simulink model "mpc_model_dual_module_tobecombined"  (R2019a)
settings: Solver=FixedStepAuto  StartTime=0.0  StopTime=Tfinal  RelTol=1e-3
values from neighbouring files (symbols this model uses):
  A = [-0.0285 -0.0014; -0.0371 -0.1476]    [model.m]
  DCLINK_Cap = 1000e-12    (= 1e-09)    [mpc_model_parameters.m]    (also in mpc_model_parameters_dual_module.m = 0.001)
  FluxPM = MeanInducedVoltagePeak/(2*pi*100)    [mpc_model_parameters.m]    (also in mpc_model_parameters_dual_module.m)
  Inertia = 1e-2    (= 0.01)    [mpc_model_parameters.m]    (also in mpc_model_parameters_dual_module.m)
  iqrated = Trated/(1.5*PolePairs*FluxPM)    [mpc_model_parameters.m]    (also in mpc_model_parameters_dual_module.m)
  Ls = 3.5e-3    (= 0.0035)    [MPC_id_iq.m]    (also in mpc_model_parameters.m = 0.00351; mpc_model_parameters_dual_module.m = 0.00343)
  M1_FaultTime = 0.25    [mpc_model_parameters_dual_module.m]
  M2_FaultTime = 20    [mpc_model_parameters_dual_module.m]
  MeanLd = (1/12)*(Module1Phase_A_Ld+Module1Phase_B_Ld+Module1Phase_C_Ld+     Module2Phase_A_Ld+Module2Phase_B_Ld+Module2Phase_C_Ld+     Module3Phase_A_Ld+Module3Phase_B_Ld+Module3Phase_C_Ld+     Module4Phase_A_Ld+Module4Phase_B_Ld+Module4Phase_C_Ld)    [mpc_model_parameters.m]    (also in mpc_model_parameters_dual_module.m)
  MeanLq = (1/12)*(Module1Phase_A_Lq+Module1Phase_B_Lq+Module1Phase_C_Lq+     Module2Phase_A_Lq+Module2Phase_B_Lq+Module2Phase_C_Lq+     Module3Phase_A_Lq+Module3Phase_B_Lq+Module3Phase_C_Lq+     Module4Phase_A_Lq+Module4Phase_B_Lq+Module4Phase_C_Lq)    [mpc_model_parameters.m]    (also in mpc_model_parameters_dual_module.m)
  PolePairs = 10    [mpc_model_parameters.m]    (also in mpc_model_parameters_dual_module.m)
  Rin = 1e-3    (= 0.001)    [mpc_model_parameters.m]    (also in mpc_model_parameters_dual_module.m)
  Rs = 0.531    [Loss_Distribution.m]    (also in MPC_id_iq.m; mpc_model_parameters.m = 0.321; mpc_model_parameters_dual_module.m = 0.539)
  Sampling_time = 1e-6    (= 1e-06)    [mpc_model_parameters.m]    (also in mpc_model_parameters_dual_module.m)
  SpeedRef1 = 50    [mpc_model_parameters.m]    (also in mpc_model_parameters_dual_module.m = 35)
  SpeedRef2 = 100    [mpc_model_parameters.m]    (also in mpc_model_parameters_dual_module.m = 35)
  SpeedRefUpdateTime = 0.25    [mpc_model_parameters.m]    (also in mpc_model_parameters_dual_module.m = 1.75)
  Tload1 = 5    [mpc_model_parameters.m]    (also in mpc_model_parameters_dual_module.m = 30)
  Tload2 = 10    [mpc_model_parameters.m]    (also in mpc_model_parameters_dual_module.m = 63.6619772368)
  TloadUpdateTime = 0.5    [mpc_model_parameters.m]    (also in mpc_model_parameters_dual_module.m)
  Vdc = 50    [mpc_model_parameters.m]    (also in mpc_model_parameters_dual_module.m = 40)
  Vin = Vdc + Rin*(Pout/Vdc)    (= 50.04)    [mpc_model_parameters.m]    (also in mpc_model_parameters_dual_module.m = 40.05)
  ViscousFriction = 1e-3    (= 0.001)    [mpc_model_parameters.m]    (also in mpc_model_parameters_dual_module.m)
undefined symbols (not defined in the file or in its folder): DiscIntNeverNeededParam
libraries: powerlib x24, dspswit3 x13, fl_lib x5, simulink x3, powerlib_meascontrol x3, nesl_utility x3, sdl_lib x1, dspsigops x1
(part 2 of 2)

== matlab function mpc_model_dual_module_tobecombined/M1_prediction ==
  data: DutyA output; DutyB output; DutyC output; iqref input; idref input; IdMeasured input; IqMeasured input; Ls input; Rs input; PolePairs input; ShaftAngularSpeed input; FluxPM input; Vdc input; ElectricalAngle input; InterruptPulse input; DutyA_prev input; DutyB_prev input; DutyC_prev input; SimulationClock input; FaultOccuranceTime input; FswSelected_prev input; FswSelected output; IqRipplePrediction output; IqRipplePrediction_prev input
function [DutyA, DutyB, DutyC, FswSelected, IqRipplePrediction]  = fcn(iqref,idref,IdMeasured, IqMeasured, Ls, Rs,PolePairs,ShaftAngularSpeed,FluxPM,Vdc,ElectricalAngle,InterruptPulse,DutyA_prev, DutyB_prev, DutyC_prev, SimulationClock,FaultOccuranceTime,FswSelected_prev, IqRipplePrediction_prev)
Ld = Ls;
Lq = Ls;
I_Normalize = 11.7362; %this is the rated value of the IqMeasured
cost = zeros(1,8);
VdPrediction_1 = zeros(1,8);
VqPrediction_1 = zeros(1,8);
% FswOptions = [5000; 10000; 15000; 20000; 25000; 30000; 35000; 40000];
FswMax = 40000;
FswOptions = 1000:1000:FswMax;
cost = zeros(1,numel(FswOptions));
VdPrediction_1 = zeros(1,numel(FswOptions));
VqPrediction_1 = zeros(1,numel(FswOptions));
IqRipplePredictionArray = zeros(1,numel(FswOptions));
VoltageDuring_T1 = zeros(1,numel(FswOptions));
VoltageDuring_T2 = zeros(1,numel(FswOptions));
VoltageDuring_T0 = zeros(1,numel(FswOptions));
MagnitudePrediction_1 = zeros(1,numel(FswOptions));

SvpwmT1Prediction_1 =  zeros(1,numel(FswOptions));
SvpwmT2Prediction_1 =  zeros(1,numel(FswOptions));
SvpwmT0Prediction_1 =  zeros(1,numel(FswOptions));

ValfaPrediction_1 = zeros(1,numel(FswOptions)); 
VbetaPrediction_1 = zeros(1,numel(FswOptions)); 
maPrediction_1 = zeros(1,numel(FswOptions)); 

IqDelta_Prediction_During_T1_1 =  zeros(1,numel(FswOptions));
IqDelta_Prediction_During_T2_1 =  zeros(1,numel(FswOptions));
IqDelta_Prediction_During_T0_1 =  zeros(1,numel(FswOptions));
VoltageVectorAnglePredictionMod_1 = zeros(1,numel(FswOptions));
VoltageVectorAnglePrediction_1 = zeros(1,numel(FswOptions));

IqRippleCoeff = 10000;
IqRefCoeff = 100000;
IdRefCoeff = 15;
FswCoeff = 1500;
if(InterruptPulse==1)
    
    for i = 1:numel(FswOptions)
        % calculate vd vq
        VdPrediction_1(i) = Rs*IdMeasured + Ld*FswOptions(i)*(idref-IdMeasured)-PolePairs*ShaftAngularSpeed*Lq*IqMeasured;
        VqPrediction_1(i) = Rs*IqMeasured + Lq*FswOptions(i)*(iqref-IqMeasured)+PolePairs*ShaftAngularSpeed*(Ld*IdMeasured+FluxPM);
        
        MagnitudePrediction_1(i) = sqrt(VdPrediction_1(i)^2+VqPrediction_1(i)^2);
        
        ValfaPrediction_1(i) = sin(ElectricalAngle)*VdPrediction_1(i)+cos(ElectricalAngle)*VqPrediction_1(i);
        VbetaPrediction_1(i) =-cos(ElectricalAngle)*VdPrediction_1(i)+sin(ElectricalAngle)*VqPrediction_1(i);     
        
        VoltageVectorAnglePrediction_1(i) = atan2(VbetaPrediction_1(i),ValfaPrediction_1(i))+4*pi;
        VoltageVectorAnglePredictionMod_1(i) = mod(VoltageVectorAnglePrediction_1(i),pi/3);
        
        maPrediction_1(i) = MagnitudePrediction_1(i)/(Vdc/sqrt(3));
        

        
        if(SimulationClock>FaultOccuranceTime)
            SvpwmT1Prediction_1(i) = (1/FswOptions(i))*maPrediction_1(i)*sin(mod(VoltageVectorAnglePrediction_1(i),pi));
            SvpwmT2Prediction_1(i) = 0;
            SvpwmT0Prediction_1(i) = (1/FswOptions(i))-SvpwmT1Prediction_1(i)-SvpwmT2Prediction_1(i);       
%             IqRippleCoeff = 0;
%             FswCoeff = 1500;
        else
            SvpwmT1Prediction_1(i) = (1/FswOptions(i))*maPrediction_1(i)*sin(pi/3-VoltageVectorAnglePredictionMod_1(i));
            SvpwmT2Prediction_1(i) = (1/FswOptions(i))*maPrediction_1(i)*sin(VoltageVectorAnglePredictionMod_1(i));
            SvpwmT0Prediction_1(i) = (1/FswOptions(i))-SvpwmT1Prediction_1(i)-SvpwmT2Prediction_1(i);    
%             IqRippleCoeff = 10000;
%             FswCoeff = 1500;
        end        
        
        VoltageDuring_T1(i) = 2/3*Vdc-MagnitudePrediction_1(i);
        VoltageDuring_T2(i) = 2/3*Vdc-MagnitudePrediction_1(i);
        VoltageDuring_T0(i) = -MagnitudePrediction_1(i);
        
        IqDelta_Prediction_During_T1_1(i) = VoltageDuring_T1(i)*SvpwmT1Prediction_1(i)/Ls;
        IqDelta_Prediction_During_T2_1(i) = VoltageDuring_T2(i)*SvpwmT2Prediction_1(i)/Ls;
        IqDelta_Prediction_During_T0_1(i) = -VoltageDuring_T0(i)*SvpwmT0Prediction_1(i)/Ls;
        
        IqRipplePredictionArray(i) = IqDelta_Prediction_During_T1_1(i)+IqDelta_Prediction_During_T2_1(i)+IqDelta_Prediction_During_T0_1(i);
        
        %predict the future output
        IdPrediction_1 = IdMeasured + (1/FswOptions(i))*(VdPrediction_1(i)/Ld-Rs/Ld*IdMeasured+Lq/Ld*PolePairs*ShaftAngularSpeed*IqMeasured);
        IqPrediction_1 = IqMeasured + (1/FswOptions(i))*(VqPrediction_1(i)*Lq-Rs/Lq*IqMeasured-Ld/Lq*PolePairs*ShaftAngularSpeed*IdMeasured-FluxPM*PolePairs*ShaftAngularSpeed/Lq);
        TePrediction_1 = 1.5*PolePairs*(FluxPM*IqPrediction_1+0*(Ld-Lq)*IdPrediction_1*IqPrediction_1); % reluctance torque component is multiplied by 0, since it caused unreasonable torque values.
        
        %calculate the cost
        if(abs(IqPrediction_1)>30)||(abs(TePrediction_1)>50)
            ProtectionConstant = inf;
        else
            ProtectionConstant = 0;
        end
        cost(i) = (IqRipplePredictionArray(i)/I_Normalize)^2*IqRippleCoeff+IqRefCoeff*((iqref-IqPrediction_1)/I_Normalize)^2+((idref-IdPrediction_1)/I_Normalize)^2*IdRefCoeff+ProtectionConstant+FswOptions(i)/FswMax*FswCoeff;%+IqRipplePrediction_prev^2*100000000;
        
    end
    
    [CostMinVal, MinimumCostIndex] = min(cost);
    
    DutyA = 0;
    DutyB = 0;
    DutyC = 0;
    VdsOptimum_1 = VdPrediction_1(MinimumCostIndex);
    VqsOptimum_1 = VqPrediction_1(MinimumCostIndex);
    FswSelected = FswOptions(MinimumCostIndex);
    

    VoltageVectorAngleOptimum = VoltageVectorAnglePrediction_1(MinimumCostIndex);
    TswSelected = 1/FswSelected;

    
    Svpwm_T1 = SvpwmT1Prediction_1(MinimumCostIndex);
    Svpwm_T2 = SvpwmT2Prediction_1(MinimumCostIndex);
    Svpwm_T0 = SvpwmT0Prediction_1(MinimumCostIndex);
    
    IqRipplePrediction = IqRipplePredictionArray(MinimumCostIndex);
    

    if(SimulationClock>FaultOccuranceTime)
        if (mod(VoltageVectorAngleOptimum, 2*pi)<=pi)  
            DutyB = (Svpwm_T1+Svpwm_T0/2)/TswSelected;
            DutyC = (Svpwm_T0/2)/TswSelected;
        else
            DutyC = (Svpwm_T1+Svpwm_T0/2)/TswSelected;
            DutyB = (Svpwm_T0/2)/TswSelected;
        end
        DutyA = 0;
        return;
    end
    
    if (mod(VoltageVectorAngleOptimum, 2*pi)<=pi/3)&&(mod(VoltageVectorAngleOptimum, 2*pi)>=0)  % sector 1
        DutyA = (Svpwm_T1+Svpwm_T2+Svpwm_T0/2)/TswSelected;
        DutyB = (Svpwm_T2+Svpwm_T0/2)/TswSelected;
        DutyC = (Svpwm_T0/2)/TswSelected;
%         sectornumber = 1;
        return;
    end
    if (mod(VoltageVectorAngleOptimum, 2*pi)<=2*pi/3)&&(mod(VoltageVectorAngleOptimum, 2*pi)>=pi/3)  % sector 2
        DutyA = (Svpwm_T1+Svpwm_T0/2)/TswSelected;
        DutyB = (Svpwm_T1+Svpwm_T2+Svpwm_T0/2)/TswSelected;
        DutyC = (Svpwm_T0/2)/TswSelected;
%         sectornumber = 2;
        return;
    end
    if (mod(VoltageVectorAngleOptimum, 2*pi)<=pi)&&(mod(VoltageVectorAngleOptimum, 2*pi)>=2*pi/3)  % sector 3
        if(mod(VoltageVectorAngleOptimum, pi)==0)
            DutyA = (Svpwm_T0/2)/TswSelected;
            DutyB = (Svpwm_T1+Svpwm_T0/2)/TswSelected;
            DutyC = (Svpwm_T1+Svpwm_T2+Svpwm_T0/2)/TswSelected;
        else
            DutyA = (Svpwm_T0/2)/TswSelected;
            DutyB = (Svpwm_T1+Svpwm_T2+Svpwm_T0/2)/TswSelected;
            DutyC = (Svpwm_T2+Svpwm_T0/2)/TswSelected;
        end
%         sectornumber = 3;
        return;
    end
    if (mod(VoltageVectorAngleOptimum, 2*pi)<=4*pi/3)&&(mod(VoltageVectorAngleOptimum, 2*pi)>=pi)  % sector 4
        DutyA = (Svpwm_T0/2)/TswSelected;
        DutyB = (Svpwm_T1+Svpwm_T0/2)/TswSelected;
        DutyC = (Svpwm_T1+Svpwm_T2+Svpwm_T0/2)/TswSelected;
%         sectornumber = 4;
        return;
    end
    if (mod(VoltageVectorAngleOptimum, 2*pi)<=5*pi/3)&&(mod(VoltageVectorAngleOptimum, 2*pi)>=4*pi/3)  % sector 5
        DutyA = (Svpwm_T2+Svpwm_T0/2)/TswSelected;
        DutyB = (Svpwm_T0/2)/TswSelected;
        DutyC = (Svpwm_T1+Svpwm_T2+Svpwm_T0/2)/TswSelected;
%         sectornumber = 5;
        return;
    end
    if (mod(VoltageVectorAngleOptimum, 2*pi)<=2*pi)&&(mod(VoltageVectorAngleOptimum, 2*pi)>=5*pi/3)  % sector 6
        DutyA = (Svpwm_T1+Svpwm_T2+Svpwm_T0/2)/TswSelected;
        DutyB = (Svpwm_T0/2)/TswSelected;
        DutyC = (Svpwm_T1+Svpwm_T0/2)/TswSelected;
%         sectornumber = 6;
        return;
    end
    
else %switching pulse
    
    FswSelected = FswSelected_prev;
    DutyA = DutyA_prev;
    DutyB = DutyB_prev;
    DutyC = DutyC_prev;
    IqRipplePrediction = IqRipplePrediction_prev;
end

== matlab function mpc_model_dual_module_tobecombined/module 2 abc to dq0 ==
  data: ids output; iqs output; ias input; ibs input; ics input; ref_frame_position input; i0 output
function [ids,iqs,i0 ]  = fcn(ias,ibs,ics,ref_frame_position)





ids = 2/3*(ias*sin(ref_frame_position)+ibs*sin(ref_frame_position-2*pi/3)+ics*sin(ref_frame_position+2*pi/3));
iqs =  2/3*(ias*cos(ref_frame_position)+ibs*cos(ref_frame_position-2*pi/3)+ics*cos(ref_frame_position+2*pi/3));
i0 = 2/3*1/2*(ias+ibs+ics);
% iqs = (vqs-fluxlinkage_qs_derivative-ref_frame_velocity*fluxlinkage_ds)/rs;
% ids = (vds-fluxlinkage_ds_derivative+ref_frame_velocity*fluxlinkage_qs)/rs;

== matlab function mpc_model_dual_module_tobecombined/prediction1 ==
  data: M2_DutyA output; M2_DutyB output; M2_DutyC output; M2_iqref_prev input; M2_idref input; M2_IdMeasured input; M2_IqMeasured input; Ls input; Rs input; PolePairs input; wref input; ShaftAngularSpeed input; ShaftAngularSpeed_prev input; FluxPM input; Vdc input; ElectricalAngle input; M2_InterruptPulse input; M2_DutyA_prev input; M2_DutyB_prev input; M2_DutyC_prev input; SimulationClock input; M2_FaultOccuranceTime input; M2_FswSelected_prev input; M2_FswSelected output; M2_IqRipplePrediction output; M2_IqRipplePrediction_prev input; M2_iqref output; M2_Speed_Error_prev input; M2_Speed_Error output
function [M2_DutyA, M2_DutyB, M2_DutyC, M2_FswSelected, M2_IqRipplePrediction,M2_iqref,M2_Speed_Error]  = fcn(M2_iqref_prev,M2_idref,M2_IdMeasured, M2_IqMeasured, Ls, Rs,PolePairs,wref, ShaftAngularSpeed,ShaftAngularSpeed_prev, FluxPM,Vdc,ElectricalAngle,M2_InterruptPulse,M2_DutyA_prev, M2_DutyB_prev, M2_DutyC_prev, SimulationClock,M2_FaultOccuranceTime,M2_FswSelected_prev, M2_IqRipplePrediction_prev,M2_Speed_Error_prev)
Ld = Ls;
Lq = Ls;
Iq_Rated = 11.7362; %this is the rated value of the M2_IqMeasured
M2_cost = zeros(1,8);
M2_VdPrediction_1 = zeros(1,8);
M2_VqPrediction_1 = zeros(1,8);
% M2_FswOptions = [5000; 10000; 15000; 20000; 25000; 30000; 35000; 40000];
M2_FswMax = 10000;
M2_FswOptions = 1000:1000:M2_FswMax;
M2_cost = zeros(1,numel(M2_FswOptions));
M2_VdPrediction_1 = zeros(1,numel(M2_FswOptions));
M2_VqPrediction_1 = zeros(1,numel(M2_FswOptions));
M2_VdPrediction_2 = zeros(1,numel(M2_FswOptions));
M2_VqPrediction_2 = zeros(1,numel(M2_FswOptions));
M2_IqRipplePredictionArray_1 = zeros(1,numel(M2_FswOptions));
M2_IqRipplePredictionArray_2 = zeros(1,numel(M2_FswOptions));
M2_VoltageDuring_T1_1 = zeros(1,numel(M2_FswOptions));
M2_VoltageDuring_T2_1 = zeros(1,numel(M2_FswOptions));
M2_VoltageDuring_T0_1 = zeros(1,numel(M2_FswOptions));
M2_VoltageDuring_T1_2 = zeros(1,numel(M2_FswOptions));
M2_VoltageDuring_T2_2 = zeros(1,numel(M2_FswOptions));
M2_VoltageDuring_T0_2 = zeros(1,numel(M2_FswOptions));
M2_MagnitudePrediction_1 = zeros(1,numel(M2_FswOptions));
M2_MagnitudePrediction_2 = zeros(1,numel(M2_FswOptions));

M2_SvpwmT1Prediction_1 =  zeros(1,numel(M2_FswOptions));
M2_SvpwmT2Prediction_1 =  zeros(1,numel(M2_FswOptions));
M2_SvpwmT0Prediction_1 =  zeros(1,numel(M2_FswOptions));

M2_SvpwmT1Prediction_2 =  zeros(1,numel(M2_FswOptions));
M2_SvpwmT2Prediction_2 =  zeros(1,numel(M2_FswOptions));
M2_SvpwmT0Prediction_2 =  zeros(1,numel(M2_FswOptions));

M2_ValfaPrediction_1 = zeros(1,numel(M2_FswOptions)); 
M2_VbetaPrediction_1 = zeros(1,numel(M2_FswOptions)); 
M2_ValfaPrediction_2 = zeros(1,numel(M2_FswOptions)); 
M2_VbetaPrediction_2 = zeros(1,numel(M2_FswOptions)); 
M2_maPrediction_1 = zeros(1,numel(M2_FswOptions)); 
M2_maPrediction_2 = zeros(1,numel(M2_FswOptions));

M2_IqDelta_Prediction_During_T1_1 =  zeros(1,numel(M2_FswOptions));
M2_IqDelta_Prediction_During_T2_1 =  zeros(1,numel(M2_FswOptions));
M2_IqDelta_Prediction_During_T0_1 =  zeros(1,numel(M2_FswOptions));
M2_IqDelta_Prediction_During_T1_2 =  zeros(1,numel(M2_FswOptions));
M2_IqDelta_Prediction_During_T2_2 =  zeros(1,numel(M2_FswOptions));
M2_IqDelta_Prediction_During_T0_2 =  zeros(1,numel(M2_FswOptions));
M2_VoltageVectorAnglePredictionMod_1 = zeros(1,numel(M2_FswOptions));
M2_VoltageVectorAnglePrediction_1 = zeros(1,numel(M2_FswOptions));
M2_VoltageVectorAnglePredictionMod_2 = zeros(1,numel(M2_FswOptions));
M2_VoltageVectorAnglePrediction_2 = zeros(1,numel(M2_FswOptions));

M2_IdPrediction_1_array = zeros(1,numel(M2_FswOptions));
M2_IqPrediction_1_array = zeros(1,numel(M2_FswOptions));
M2_IdPrediction_2_array = zeros(1,numel(M2_FswOptions));
M2_IqPrediction_2_array = zeros(1,numel(M2_FswOptions));

M2_MinimumCostValue = 1e20;
M2_MinimumCostIndex = -1;

M2_IqRippleCoeff = 100000;
M2_IqRefCoeff = 10000;
M2_IdRefCoeff = 15;
M2_FswCoeff = 1250;
M2_Iq_1_Method1 = 0;
M2_Id_1_Method1 = 0;
M2_Iq_2_Method1 = 0;
M2_Id_2_Method1 = 0;
M2_Kp = 0.35;
M2_Ki = 10;
M2_Ts_PI = 1/40000;
% y = y_prev + Kp*(u-u_prev)+Ts/2*Ki*(u+u_prev);
if(M2_InterruptPulse==1)
    M2_Speed_Error =  wref-ShaftAngularSpeed;
    
    M2_iqref = M2_iqref_prev + M2_Kp*(M2_Speed_Error-M2_Speed_Error_prev)+M2_Ts_PI/2*M2_Ki*((M2_Speed_Error+M2_Speed_Error_prev));
    if(abs(M2_iqref)>(2*Iq_Rated))
        if(M2_iqref>0)
            M2_iqref = (2*Iq_Rated);
        else
            M2_iqref = -(2*Iq_Rated);
        end
    end
    for i = 1:numel(M2_FswOptions)
        %% first prediction
        M2_VdPrediction_1(i) = Rs*M2_IdMeasured + Ld*M2_FswOptions(i)*(M2_idref-M2_IdMeasured)-PolePairs*ShaftAngularSpeed*Lq*M2_IqMeasured;
        M2_VqPrediction_1(i) = Rs*M2_IqMeasured + Lq*M2_FswOptions(i)*(M2_iqref-M2_IqMeasured)+PolePairs*ShaftAngularSpeed*(Ld*M2_IdMeasured+FluxPM);
        
%         MagnitudePrediction_1(i) = sqrt(M2_VdPrediction_1(i)^2+M2_VqPrediction_1(i)^2);
%         
%         ValfaPrediction_1(i) = sin(ElectricalAngle)*M2_VdPrediction_1(i)+cos(ElectricalAngle)*M2_VqPrediction_1(i);
%         VbetaPrediction_1(i) =-cos(ElectricalAngle)*M2_VdPrediction_1(i)+sin(ElectricalAngle)*M2_VqPrediction_1(i);     
%         
%         VoltageVectorAnglePrediction_1(i) = atan2(VbetaPrediction_1(i),ValfaPrediction_1(i))+4*pi;
%         VoltageVectorAnglePredictionMod_1(i) = mod(VoltageVectorAnglePrediction_1(i),pi/3);
%         
%         maPrediction_1(i) = MagnitudePrediction_1(i)/(Vdc/sqrt(3));
%         
%         SvpwmT1Prediction_1(i) = (1/M2_FswOptions(i))*maPrediction_1(i)*sin(pi/3-VoltageVectorAnglePredictionMod_1(i));
%         SvpwmT2Prediction_1(i) = (1/M2_FswOptions(i))*maPrediction_1(i)*sin(VoltageVectorAnglePredictionMod_1(i));
%         SvpwmT0Prediction_1(i) = (1/M2_FswOptions(i))-SvpwmT1Prediction_1(i)-SvpwmT2Prediction_1(i);        
%         
%         VoltageDuring_T1_1(i) = 2/3*Vdc-MagnitudePrediction_1(i);
%         VoltageDuring_T2_1(i) = 2/3*Vdc-MagnitudePrediction_1(i);
%         VoltageDuring_T0_1(i) = -MagnitudePrediction_1(i);
%         
%         IqDelta_Prediction_During_T1_1(i) = VoltageDuring_T1_1(i)*SvpwmT1Prediction_1(i)/Ls;
%         IqDelta_Prediction_During_T2_1(i) = VoltageDuring_T2_1(i)*SvpwmT2Prediction_1(i)/Ls;
%         IqDelta_Prediction_During_T0_1(i) = -VoltageDuring_T0_1(i)*SvpwmT0Prediction_1(i)/Ls;
%         
%         IqRipplePredictionArray_1(i) = IqDelta_Prediction_During_T1_1(i)+IqDelta_Prediction_During_T2_1(i)+IqDelta_Prediction_During_T0_1(i);
        
        %predict the future output
        M2_IdPrediction_1 = M2_IdMeasured + (1/M2_FswOptions(i))*(M2_VdPrediction_1(i)/Ld-Rs/Ld*M2_IdMeasured+Lq/Ld*PolePairs*ShaftAngularSpeed*M2_IqMeasured);
        M2_IqPrediction_1 = M2_IqMeasured + (1/M2_FswOptions(i))*(M2_VqPrediction_1(i)/Lq-Rs/Lq*M2_IqMeasured-Ld/Lq*PolePairs*ShaftAngularSpeed*M2_IdMeasured-FluxPM*PolePairs*ShaftAngularSpeed/Lq);
        M2_VqPrediction_1 = 1.5*PolePairs*(FluxPM*M2_IqPrediction_1+0*(Ld-Lq)*M2_IdPrediction_1*M2_IqPrediction_1); % reluctance torque component is multiplied by 0, since it caused unreasonable torque values.
                
        M2_IdPrediction_1_array(i) = M2_IdPrediction_1;
        M2_IqPrediction_1_array(i) = M2_IqPrediction_1;
        
        %% second prediction
        M2_VdPrediction_2(i) = Rs*M2_IdPrediction_1 + Ld*M2_FswOptions(i)*(idref-M2_IdMeasured)-PolePairs*ShaftAngularSpeed*Lq*M2_IqPrediction_1;
        M2_VqPrediction_2(i) = Rs*M2_IqPrediction_1 + Lq*M2_FswOptions(i)*(M2_iqref-M2_IqMeasured)+PolePairs*ShaftAngularSpeed*(Ld*M2_IdPrediction_1+FluxPM);        
        
        M2_MagnitudePrediction_2(i) = sqrt(M2_VdPrediction_2(i)^2+M2_VqPrediction_2(i)^2);
        
        M2_ValfaPrediction_2(i) = sin(ElectricalAngle)*M2_VdPrediction_2(i)+cos(ElectricalAngle)*M2_VqPrediction_2(i);
        M2_VbetaPrediction_2(i) =-cos(ElectricalAngle)*M2_VdPrediction_2(i)+sin(ElectricalAngle)*M2_VqPrediction_2(i);      
        
        M2_VoltageVectorAnglePrediction_2(i) = atan2(M2_VbetaPrediction_2(i),M2_ValfaPrediction_2(i))+4*pi;
        M2_VoltageVectorAnglePredictionMod_2(i) = mod(M2_VoltageVectorAnglePrediction_2(i),pi/3);   
        
        M2_maPrediction_2(i) = M2_MagnitudePrediction_2(i)/(Vdc/sqrt(3)); 
        
        M2_SvpwmT1Prediction_2(i) = (1/M2_FswOptions(i))*M2_maPrediction_2(i)*sin(pi/3-M2_VoltageVectorAnglePredictionMod_2(i));
        M2_SvpwmT2Prediction_2(i) = (1/M2_FswOptions(i))*M2_maPrediction_2(i)*sin(M2_VoltageVectorAnglePredictionMod_2(i));
        M2_SvpwmT0Prediction_2(i) = (1/M2_FswOptions(i))-M2_SvpwmT1Prediction_2(i)-M2_SvpwmT2Prediction_2(i); 
        
        M2_VoltageDuring_T1_2(i) = 2/3*Vdc-M2_MagnitudePrediction_2(i);
        M2_VoltageDuring_T2_2(i) = 2/3*Vdc-M2_MagnitudePrediction_2(i);
        M2_VoltageDuring_T0_2(i) = -M2_MagnitudePrediction_2(i);
        
        M2_IqDelta_Prediction_During_T1_2(i) = M2_VoltageDuring_T1_2(i)*M2_SvpwmT1Prediction_2(i)/Ls;
        M2_IqDelta_Prediction_During_T2_2(i) = M2_VoltageDuring_T2_2(i)*M2_SvpwmT2Prediction_2(i)/Ls;
        M2_IqDelta_Prediction_During_T0_2(i) = -M2_VoltageDuring_T0_2(i)*M2_SvpwmT0Prediction_2(i)/Ls;        
        
        M2_IqRipplePredictionArray_2(i) = M2_IqDelta_Prediction_During_T1_2(i)+M2_IqDelta_Prediction_During_T2_2(i)+M2_IqDelta_Prediction_During_T0_2(i);
        
        M2_IdPrediction_2 = M2_IdPrediction_1 + (1/M2_FswOptions(i))*(M2_VdPrediction_2(i)/Ld-Rs/Ld*M2_IdPrediction_1+Lq/Ld*PolePairs*ShaftAngularSpeed*M2_IqPrediction_1);
        M2_IqPrediction_2 = M2_IqPrediction_1 + (1/M2_FswOptions(i))*(M2_VqPrediction_2(i)/Lq-Rs/Lq*M2_IqPrediction_1-Ld/Lq*PolePairs*ShaftAngularSpeed*M2_IdPrediction_1-FluxPM*PolePairs*ShaftAngularSpeed/Lq);                
        
        M2_IdPrediction_2_array(i) = M2_IdPrediction_2;
        M2_IqPrediction_2_array(i) = M2_IqPrediction_2;
        
        %% calculate the M2_cost
        if(abs(M2_IqPrediction_1)>30)||(abs(M2_VqPrediction_1)>50)
            M2_ProtectionConstant = inf;
        else
            M2_ProtectionConstant = 0;
        end
%         M2_cost(i) = (IqRipplePredictionArray_1(i)/Iq_Rated)^2*M2_IqRippleCoeff+IqRefCoeff*((M2_iqref-M2_IqPrediction_1)/Iq_Rated)^2+((idref-M2_IdPrediction_1)/Iq_Rated)^2*IdRefCoeff+M2_ProtectionConstant+M2_FswOptions(i)/M2_FswMax*FswCoeff;%+M2_IqRipplePrediction_prev^2*100000000;
        M2_cost(i) = (M2_IqRipplePredictionArray_2(i)/Iq_Rated)^2*M2_IqRippleCoeff+M2_IqRefCoeff*((M2_iqref-M2_IqPrediction_2)/Iq_Rated)^2+((M2_idref-M2_IdPrediction_2)/Iq_Rated)^2*M2_IdRefCoeff+M2_ProtectionConstant+M2_FswOptions(i)/M2_FswMax*M2_FswCoeff;%+M2_IqRipplePrediction_prev^2*100000000;
        if(M2_cost(i)<M2_MinimumCostValue)
            M2_MinimumCostValue = M2_cost(i);
            M2_MinimumCostIndex = i;
        end
        
    end
    
%     [CostMinVal, M2_MinimumCostIndex] = min(M2_cost);
    
    M2_DutyA = 0;
    M2_DutyB = 0;
    M2_DutyC = 0;
    M2_VdsOptimum_1 = M2_VdPrediction_2(M2_MinimumCostIndex);
    M2_VqsOptimum_1 = M2_VqPrediction_2(M2_MinimumCostIndex);
    M2_FswSelected = M2_FswOptions(M2_MinimumCostIndex);
    
    M2_Iq_1_Method1 = M2_IqPrediction_1_array(M2_MinimumCostIndex);
    M2_Id_1_Method1 = M2_IdPrediction_1_array(M2_MinimumCostIndex);

    M2_Iq_2_Method1 = M2_IqPrediction_2_array(M2_MinimumCostIndex);
    M2_Id_2_Method1 = M2_IdPrediction_2_array(M2_MinimumCostIndex);
    
    M2_VoltageVectorAngleOptimum = M2_VoltageVectorAnglePrediction_2(M2_MinimumCostIndex);
    M2_TswSelected = 1/M2_FswSelected;

    
    M2_Svpwm_T1 = M2_SvpwmT1Prediction_2(M2_MinimumCostIndex);
    M2_Svpwm_T2 = M2_SvpwmT2Prediction_2(M2_MinimumCostIndex);
    M2_Svpwm_T0 = M2_SvpwmT0Prediction_2(M2_MinimumCostIndex);
    
    M2_IqRipplePrediction = M2_IqRipplePredictionArray_2(M2_MinimumCostIndex);
    
    if (mod(M2_VoltageVectorAngleOptimum, 2*pi)<=pi/3)&&(mod(M2_VoltageVectorAngleOptimum, 2*pi)>=0)  % sector 1
        M2_DutyA = (M2_Svpwm_T1+M2_Svpwm_T2+M2_Svpwm_T0/2)/M2_TswSelected;
        M2_DutyB = (M2_Svpwm_T2+M2_Svpwm_T0/2)/M2_TswSelected;
        M2_DutyC = (M2_Svpwm_T0/2)/M2_TswSelected;
%         sectornumber = 1;
        return;
    end
    if (mod(M2_VoltageVectorAngleOptimum, 2*pi)<=2*pi/3)&&(mod(M2_VoltageVectorAngleOptimum, 2*pi)>=pi/3)  % sector 2
        M2_DutyA = (M2_Svpwm_T1+M2_Svpwm_T0/2)/M2_TswSelected;
        M2_DutyB = (M2_Svpwm_T1+M2_Svpwm_T2+M2_Svpwm_T0/2)/M2_TswSelected;
        M2_DutyC = (M2_Svpwm_T0/2)/M2_TswSelected;
%         sectornumber = 2;
        return;
    end
    if (mod(M2_VoltageVectorAngleOptimum, 2*pi)<=pi)&&(mod(M2_VoltageVectorAngleOptimum, 2*pi)>=2*pi/3)  % sector 3
        if(mod(M2_VoltageVectorAngleOptimum, pi)==0)
            M2_DutyA = (M2_Svpwm_T0/2)/M2_TswSelected;
            M2_DutyB = (M2_Svpwm_T1+M2_Svpwm_T0/2)/M2_TswSelected;
            M2_DutyC = (M2_Svpwm_T1+M2_Svpwm_T2+M2_Svpwm_T0/2)/M2_TswSelected;
        else
            M2_DutyA = (M2_Svpwm_T0/2)/M2_TswSelected;
            M2_DutyB = (M2_Svpwm_T1+M2_Svpwm_T2+M2_Svpwm_T0/2)/M2_TswSelected;
            M2_DutyC = (M2_Svpwm_T2+M2_Svpwm_T0/2)/M2_TswSelected;
        end
%         sectornumber = 3;
        return;
    end
    if (mod(M2_VoltageVectorAngleOptimum, 2*pi)<=4*pi/3)&&(mod(M2_VoltageVectorAngleOptimum, 2*pi)>=pi)  % sector 4
        M2_DutyA = (M2_Svpwm_T0/2)/M2_TswSelected;
        M2_DutyB = (M2_Svpwm_T1+M2_Svpwm_T0/2)/M2_TswSelected;
        M2_DutyC = (M2_Svpwm_T1+M2_Svpwm_T2+M2_Svpwm_T0/2)/M2_TswSelected;
%         sectornumber = 4;
        return;
    end
    if (mod(M2_VoltageVectorAngleOptimum, 2*pi)<=5*pi/3)&&(mod(M2_VoltageVectorAngleOptimum, 2*pi)>=4*pi/3)  % sector 5
        M2_DutyA = (M2_Svpwm_T2+M2_Svpwm_T0/2)/M2_TswSelected;
        M2_DutyB = (M2_Svpwm_T0/2)/M2_TswSelected;
        M2_DutyC = (M2_Svpwm_T1+M2_Svpwm_T2+M2_Svpwm_T0/2)/M2_TswSelected;
%         sectornumber = 5;
        return;
    end
    if (mod(M2_VoltageVectorAngleOptimum, 2*pi)<=2*pi)&&(mod(M2_VoltageVectorAngleOptimum, 2*pi)>=5*pi/3)  % sector 6
        M2_DutyA = (M2_Svpwm_T1+M2_Svpwm_T2+M2_Svpwm_T0/2)/M2_TswSelected;
        M2_DutyB = (M2_Svpwm_T0/2)/M2_TswSelected;
        M2_DutyC = (M2_Svpwm_T1+M2_Svpwm_T0/2)/M2_TswSelected;
%         sectornumber = 6;
        return;
    end
    
else %switching pulse
    M2_iqref = M2_iqref_prev;
    M2_Speed_Error = M2_Speed_Error_prev;
    M2_FswSelected = M2_FswSelected_prev;
    M2_DutyA = M2_DutyA_prev;
    M2_DutyB = M2_DutyB_prev;
    M2_DutyC = M2_DutyC_prev;
    M2_IqRipplePrediction = M2_IqRipplePrediction_prev;
end

== matlab function mpc_model_dual_module_tobecombined/module 1 abc to dq0 ==
  data: ids output; iqs output; ias input; ibs input; ics input; ref_frame_position input; i0 output
function [ids,iqs,i0 ]  = fcn(ias,ibs,ics,ref_frame_position)





ids = 2/3*(ias*sin(ref_frame_position)+ibs*sin(ref_frame_position-2*pi/3)+ics*sin(ref_frame_position+2*pi/3));
iqs =  2/3*(ias*cos(ref_frame_position)+ibs*cos(ref_frame_position-2*pi/3)+ics*cos(ref_frame_position+2*pi/3));
i0 = 2/3*1/2*(ias+ibs+ics);
% iqs = (vqs-fluxlinkage_qs_derivative-ref_frame_velocity*fluxlinkage_ds)/rs;
% ids = (vds-fluxlinkage_ds_derivative+ref_frame_velocity*fluxlinkage_qs)/rs;

== matlab function mpc_model_dual_module_tobecombined/prediction ==
  data: M1_DutyA output; M1_DutyB output; M1_DutyC output; M1_iqref_prev input; M1_idref input; M1_IdMeasured input; M1_IqMeasured input; Ls input; Rs input; PolePairs input; wref input; ShaftAngularSpeed input; ShaftAngularSpeed_prev input; FluxPM input; Vdc input; ElectricalAngle input; M1_InterruptPulse input; M1_DutyA_prev input; M1_DutyB_prev input; M1_DutyC_prev input; SimulationClock input; M1_FaultOccuranceTime input; M1_FswSelected_prev input; M1_FswSelected output; M1_IqRipplePrediction output; M1_IqRipplePrediction_prev input; M1_iqref output; M1_Speed_Error_prev input; M1_Speed_Error output
function [M1_DutyA, M1_DutyB, M1_DutyC, M1_FswSelected, M1_IqRipplePrediction,M1_iqref,M1_Speed_Error]  = fcn(M1_iqref_prev,M1_idref,M1_IdMeasured, M1_IqMeasured, Ls, Rs,PolePairs,wref, ShaftAngularSpeed,ShaftAngularSpeed_prev, FluxPM,Vdc,ElectricalAngle,M1_InterruptPulse,M1_DutyA_prev, M1_DutyB_prev, M1_DutyC_prev, SimulationClock,M1_FaultOccuranceTime,M1_FswSelected_prev, M1_IqRipplePrediction_prev,M1_Speed_Error_prev)
Ld = Ls;
Lq = Ls;
Iq_Rated = 11.7362; %this is the rated value of the M1_IqMeasured
M1_cost = zeros(1,8);
M1_VdPrediction_1 = zeros(1,8);
M1_VqPrediction_1 = zeros(1,8);
% M1_FswOptions = [5000; 10000; 15000; 20000; 25000; 30000; 35000; 40000];
M1_FswMax = 10000;
M1_FswOptions = 1000:1000:M1_FswMax;
M1_cost = zeros(1,numel(M1_FswOptions));
M1_VdPrediction_1 = zeros(1,numel(M1_FswOptions));
M1_VqPrediction_1 = zeros(1,numel(M1_FswOptions));
M1_VdPrediction_2 = zeros(1,numel(M1_FswOptions));
M1_VqPrediction_2 = zeros(1,numel(M1_FswOptions));
M1_IqRipplePredictionArray_1 = zeros(1,numel(M1_FswOptions));
M1_IqRipplePredictionArray_2 = zeros(1,numel(M1_FswOptions));
M1_VoltageDuring_T1_1 = zeros(1,numel(M1_FswOptions));
M1_VoltageDuring_T2_1 = zeros(1,numel(M1_FswOptions));
M1_VoltageDuring_T0_1 = zeros(1,numel(M1_FswOptions));
M1_VoltageDuring_T1_2 = zeros(1,numel(M1_FswOptions));
M1_VoltageDuring_T2_2 = zeros(1,numel(M1_FswOptions));
M1_VoltageDuring_T0_2 = zeros(1,numel(M1_FswOptions));
M1_MagnitudePrediction_1 = zeros(1,numel(M1_FswOptions));
M1_MagnitudePrediction_2 = zeros(1,numel(M1_FswOptions));

M1_SvpwmT1Prediction_1 =  zeros(1,numel(M1_FswOptions));
M1_SvpwmT2Prediction_1 =  zeros(1,numel(M1_FswOptions));
M1_SvpwmT0Prediction_1 =  zeros(1,numel(M1_FswOptions));

M1_SvpwmT1Prediction_2 =  zeros(1,numel(M1_FswOptions));
M1_SvpwmT2Prediction_2 =  zeros(1,numel(M1_FswOptions));
M1_SvpwmT0Prediction_2 =  zeros(1,numel(M1_FswOptions));

M1_ValfaPrediction_1 = zeros(1,numel(M1_FswOptions)); 
M1_VbetaPrediction_1 = zeros(1,numel(M1_FswOptions)); 
M1_ValfaPrediction_2 = zeros(1,numel(M1_FswOptions)); 
M1_VbetaPrediction_2 = zeros(1,numel(M1_FswOptions)); 
M1_maPrediction_1 = zeros(1,numel(M1_FswOptions)); 
M1_maPrediction_2 = zeros(1,numel(M1_FswOptions));

M1_IqDelta_Prediction_During_T1_1 =  zeros(1,numel(M1_FswOptions));
M1_IqDelta_Prediction_During_T2_1 =  zeros(1,numel(M1_FswOptions));
M1_IqDelta_Prediction_During_T0_1 =  zeros(1,numel(M1_FswOptions));
M1_IqDelta_Prediction_During_T1_2 =  zeros(1,numel(M1_FswOptions));
M1_IqDelta_Prediction_During_T2_2 =  zeros(1,numel(M1_FswOptions));
M1_IqDelta_Prediction_During_T0_2 =  zeros(1,numel(M1_FswOptions));
M1_VoltageVectorAnglePredictionMod_1 = zeros(1,numel(M1_FswOptions));
M1_VoltageVectorAnglePrediction_1 = zeros(1,numel(M1_FswOptions));
M1_VoltageVectorAnglePredictionMod_2 = zeros(1,numel(M1_FswOptions));
M1_VoltageVectorAnglePrediction_2 = zeros(1,numel(M1_FswOptions));

M1_IdPrediction_1_array = zeros(1,numel(M1_FswOptions));
M1_IqPrediction_1_array = zeros(1,numel(M1_FswOptions));
M1_IdPrediction_2_array = zeros(1,numel(M1_FswOptions));
M1_IqPrediction_2_array = zeros(1,numel(M1_FswOptions));

M1_MinimumCostValue = 1e20;
M1_MinimumCostIndex = -1;

M1_IqRippleCoeff = 100000;
M1_IqRefCoeff = 10000;
M1_IdRefCoeff = 15;
M1_FswCoeff = 1250;
M1_Iq_1_Method1 = 0;
M1_Id_1_Method1 = 0;
M1_Iq_2_Method1 = 0;
M1_Id_2_Method1 = 0;
M1_Kp = 0.35;
M1_Ki = 10;
M1_Ts_PI = 1/40000;
% y = y_prev + Kp*(u-u_prev)+Ts/2*Ki*(u+u_prev);
if(M1_InterruptPulse==1)
    M1_Speed_Error =  wref-ShaftAngularSpeed;
    
    M1_iqref = M1_iqref_prev + M1_Kp*(M1_Speed_Error-M1_Speed_Error_prev)+M1_Ts_PI/2*M1_Ki*((M1_Speed_Error+M1_Speed_Error_prev));
    if(abs(M1_iqref)>(2*Iq_Rated))
        if(M1_iqref>0)
            M1_iqref = (2*Iq_Rated);
        else
            M1_iqref = -(2*Iq_Rated);
        end
    end
    for i = 1:numel(M1_FswOptions)
        %% first prediction
        M1_VdPrediction_1(i) = Rs*M1_IdMeasured + Ld*M1_FswOptions(i)*(M1_idref-M1_IdMeasured)-PolePairs*ShaftAngularSpeed*Lq*M1_IqMeasured;
        M1_VqPrediction_1(i) = Rs*M1_IqMeasured + Lq*M1_FswOptions(i)*(M1_iqref-M1_IqMeasured)+PolePairs*ShaftAngularSpeed*(Ld*M1_IdMeasured+FluxPM);
        
%         MagnitudePrediction_1(i) = sqrt(M1_VdPrediction_1(i)^2+M1_VqPrediction_1(i)^2);
%         
%         ValfaPrediction_1(i) = sin(ElectricalAngle)*M1_VdPrediction_1(i)+cos(ElectricalAngle)*M1_VqPrediction_1(i);
%         VbetaPrediction_1(i) =-cos(ElectricalAngle)*M1_VdPrediction_1(i)+sin(ElectricalAngle)*M1_VqPrediction_1(i);     
%         
%         VoltageVectorAnglePrediction_1(i) = atan2(VbetaPrediction_1(i),ValfaPrediction_1(i))+4*pi;
%         VoltageVectorAnglePredictionMod_1(i) = mod(VoltageVectorAnglePrediction_1(i),pi/3);
%         
%         maPrediction_1(i) = MagnitudePrediction_1(i)/(Vdc/sqrt(3));
%         
%         SvpwmT1Prediction_1(i) = (1/M1_FswOptions(i))*maPrediction_1(i)*sin(pi/3-VoltageVectorAnglePredictionMod_1(i));
%         SvpwmT2Prediction_1(i) = (1/M1_FswOptions(i))*maPrediction_1(i)*sin(VoltageVectorAnglePredictionMod_1(i));
%         SvpwmT0Prediction_1(i) = (1/M1_FswOptions(i))-SvpwmT1Prediction_1(i)-SvpwmT2Prediction_1(i);        
%         
%         VoltageDuring_T1_1(i) = 2/3*Vdc-MagnitudePrediction_1(i);
%         VoltageDuring_T2_1(i) = 2/3*Vdc-MagnitudePrediction_1(i);
%         VoltageDuring_T0_1(i) = -MagnitudePrediction_1(i);
%         
%         IqDelta_Prediction_During_T1_1(i) = VoltageDuring_T1_1(i)*SvpwmT1Prediction_1(i)/Ls;
%         IqDelta_Prediction_During_T2_1(i) = VoltageDuring_T2_1(i)*SvpwmT2Prediction_1(i)/Ls;
%         IqDelta_Prediction_During_T0_1(i) = -VoltageDuring_T0_1(i)*SvpwmT0Prediction_1(i)/Ls;
%         
%         IqRipplePredictionArray_1(i) = IqDelta_Prediction_During_T1_1(i)+IqDelta_Prediction_During_T2_1(i)+IqDelta_Prediction_During_T0_1(i);
        
        %predict the future output
        M1_IdPrediction_1 = M1_IdMeasured + (1/M1_FswOptions(i))*(M1_VdPrediction_1(i)/Ld-Rs/Ld*M1_IdMeasured+Lq/Ld*PolePairs*ShaftAngularSpeed*M1_IqMeasured);
        M1_IqPrediction_1 = M1_IqMeasured + (1/M1_FswOptions(i))*(M1_VqPrediction_1(i)/Lq-Rs/Lq*M1_IqMeasured-Ld/Lq*PolePairs*ShaftAngularSpeed*M1_IdMeasured-FluxPM*PolePairs*ShaftAngularSpeed/Lq);
        M1_VqPrediction_1 = 1.5*PolePairs*(FluxPM*M1_IqPrediction_1+0*(Ld-Lq)*M1_IdPrediction_1*M1_IqPrediction_1); % reluctance torque component is multiplied by 0, since it caused unreasonable torque values.
                
        M1_IdPrediction_1_array(i) = M1_IdPrediction_1;
        M1_IqPrediction_1_array(i) = M1_IqPrediction_1;
        
        %% second prediction
        M1_VdPrediction_2(i) = Rs*M1_IdPrediction_1 + Ld*M1_FswOptions(i)*(idref-M1_IdMeasured)-PolePairs*ShaftAngularSpeed*Lq*M1_IqPrediction_1;
        M1_VqPrediction_2(i) = Rs*M1_IqPrediction_1 + Lq*M1_FswOptions(i)*(M1_iqref-M1_IqMeasured)+PolePairs*ShaftAngularSpeed*(Ld*M1_IdPrediction_1+FluxPM);        
        
        M1_MagnitudePrediction_2(i) = sqrt(M1_VdPrediction_2(i)^2+M1_VqPrediction_2(i)^2);
        
        M1_ValfaPrediction_2(i) = sin(ElectricalAngle)*M1_VdPrediction_2(i)+cos(ElectricalAngle)*M1_VqPrediction_2(i);
        M1_VbetaPrediction_2(i) =-cos(ElectricalAngle)*M1_VdPrediction_2(i)+sin(ElectricalAngle)*M1_VqPrediction_2(i);      
        
        M1_VoltageVectorAnglePrediction_2(i) = atan2(M1_VbetaPrediction_2(i),M1_ValfaPrediction_2(i))+4*pi;
        M1_VoltageVectorAnglePredictionMod_2(i) = mod(M1_VoltageVectorAnglePrediction_2(i),pi/3);   
        
        M1_maPrediction_2(i) = M1_MagnitudePrediction_2(i)/(Vdc/sqrt(3)); 
        
        M1_SvpwmT1Prediction_2(i) = (1/M1_FswOptions(i))*M1_maPrediction_2(i)*sin(pi/3-M1_VoltageVectorAnglePredictionMod_2(i));
        M1_SvpwmT2Prediction_2(i) = (1/M1_FswOptions(i))*M1_maPrediction_2(i)*sin(M1_VoltageVectorAnglePredictionMod_2(i));
        M1_SvpwmT0Prediction_2(i) = (1/M1_FswOptions(i))-M1_SvpwmT1Prediction_2(i)-M1_SvpwmT2Prediction_2(i); 
        
        M1_VoltageDuring_T1_2(i) = 2/3*Vdc-M1_MagnitudePrediction_2(i);
        M1_VoltageDuring_T2_2(i) = 2/3*Vdc-M1_MagnitudePrediction_2(i);
        M1_VoltageDuring_T0_2(i) = -M1_MagnitudePrediction_2(i);
        
        M1_IqDelta_Prediction_During_T1_2(i) = M1_VoltageDuring_T1_2(i)*M1_SvpwmT1Prediction_2(i)/Ls;
        M1_IqDelta_Prediction_During_T2_2(i) = M1_VoltageDuring_T2_2(i)*M1_SvpwmT2Prediction_2(i)/Ls;
        M1_IqDelta_Prediction_During_T0_2(i) = -M1_VoltageDuring_T0_2(i)*M1_SvpwmT0Prediction_2(i)/Ls;        
        
        M1_IqRipplePredictionArray_2(i) = M1_IqDelta_Prediction_During_T1_2(i)+M1_IqDelta_Prediction_During_T2_2(i)+M1_IqDelta_Prediction_During_T0_2(i);
        
        M1_IdPrediction_2 = M1_IdPrediction_1 + (1/M1_FswOptions(i))*(M1_VdPrediction_2(i)/Ld-Rs/Ld*M1_IdPrediction_1+Lq/Ld*PolePairs*ShaftAngularSpeed*M1_IqPrediction_1);
        M1_IqPrediction_2 = M1_IqPrediction_1 + (1/M1_FswOptions(i))*(M1_VqPrediction_2(i)/Lq-Rs/Lq*M1_IqPrediction_1-Ld/Lq*PolePairs*ShaftAngularSpeed*M1_IdPrediction_1-FluxPM*PolePairs*ShaftAngularSpeed/Lq);                
        
        M1_IdPrediction_2_array(i) = M1_IdPrediction_2;
        M1_IqPrediction_2_array(i) = M1_IqPrediction_2;
        
        %% calculate the M1_cost
        if(abs(M1_IqPrediction_1)>30)||(abs(M1_VqPrediction_1)>50)
            M1_ProtectionConstant = inf;
        else
            M1_ProtectionConstant = 0;
        end
%         M1_cost(i) = (IqRipplePredictionArray_1(i)/Iq_Rated)^2*M1_IqRippleCoeff+IqRefCoeff*((M1_iqref-M1_IqPrediction_1)/Iq_Rated)^2+((idref-M1_IdPrediction_1)/Iq_Rated)^2*IdRefCoeff+M1_ProtectionConstant+M1_FswOptions(i)/M1_FswMax*FswCoeff;%+M1_IqRipplePrediction_prev^2*100000000;
        M1_cost(i) = (M1_IqRipplePredictionArray_2(i)/Iq_Rated)^2*M1_IqRippleCoeff+M1_IqRefCoeff*((M1_iqref-M1_IqPrediction_2)/Iq_Rated)^2+((M1_idref-M1_IdPrediction_2)/Iq_Rated)^2*M1_IdRefCoeff+M1_ProtectionConstant+M1_FswOptions(i)/M1_FswMax*M1_FswCoeff;%+M1_IqRipplePrediction_prev^2*100000000;
        if(M1_cost(i)<M1_MinimumCostValue)
            M1_MinimumCostValue = M1_cost(i);
            M1_MinimumCostIndex = i;
        end
        
    end
    
%     [CostMinVal, M1_MinimumCostIndex] = min(M1_cost);
    
    M1_DutyA = 0;
    M1_DutyB = 0;
    M1_DutyC = 0;
    M1_VdsOptimum_1 = M1_VdPrediction_2(M1_MinimumCostIndex);
    M1_VqsOptimum_1 = M1_VqPrediction_2(M1_MinimumCostIndex);
    M1_FswSelected = M1_FswOptions(M1_MinimumCostIndex);
    
    M1_Iq_1_Method1 = M1_IqPrediction_1_array(M1_MinimumCostIndex);
    M1_Id_1_Method1 = M1_IdPrediction_1_array(M1_MinimumCostIndex);

    M1_Iq_2_Method1 = M1_IqPrediction_2_array(M1_MinimumCostIndex);
    M1_Id_2_Method1 = M1_IdPrediction_2_array(M1_MinimumCostIndex);
    
    M1_VoltageVectorAngleOptimum = M1_VoltageVectorAnglePrediction_2(M1_MinimumCostIndex);
    M1_TswSelected = 1/M1_FswSelected;

    
    M1_Svpwm_T1 = M1_SvpwmT1Prediction_2(M1_MinimumCostIndex);
    M1_Svpwm_T2 = M1_SvpwmT2Prediction_2(M1_MinimumCostIndex);
    M1_Svpwm_T0 = M1_SvpwmT0Prediction_2(M1_MinimumCostIndex);
    
    M1_IqRipplePrediction = M1_IqRipplePredictionArray_2(M1_MinimumCostIndex);
    
    if (mod(M1_VoltageVectorAngleOptimum, 2*pi)<=pi/3)&&(mod(M1_VoltageVectorAngleOptimum, 2*pi)>=0)  % sector 1
        M1_DutyA = (M1_Svpwm_T1+M1_Svpwm_T2+M1_Svpwm_T0/2)/M1_TswSelected;
        M1_DutyB = (M1_Svpwm_T2+M1_Svpwm_T0/2)/M1_TswSelected;
        M1_DutyC = (M1_Svpwm_T0/2)/M1_TswSelected;
%         sectornumber = 1;
        return;
    end
    if (mod(M1_VoltageVectorAngleOptimum, 2*pi)<=2*pi/3)&&(mod(M1_VoltageVectorAngleOptimum, 2*pi)>=pi/3)  % sector 2
        M1_DutyA = (M1_Svpwm_T1+M1_Svpwm_T0/2)/M1_TswSelected;
        M1_DutyB = (M1_Svpwm_T1+M1_Svpwm_T2+M1_Svpwm_T0/2)/M1_TswSelected;
        M1_DutyC = (M1_Svpwm_T0/2)/M1_TswSelected;
%         sectornumber = 2;
        return;
    end
    if (mod(M1_VoltageVectorAngleOptimum, 2*pi)<=pi)&&(mod(M1_VoltageVectorAngleOptimum, 2*pi)>=2*pi/3)  % sector 3
        if(mod(M1_VoltageVectorAngleOptimum, pi)==0)
            M1_DutyA = (M1_Svpwm_T0/2)/M1_TswSelected;
            M1_DutyB = (M1_Svpwm_T1+M1_Svpwm_T0/2)/M1_TswSelected;
            M1_DutyC = (M1_Svpwm_T1+M1_Svpwm_T2+M1_Svpwm_T0/2)/M1_TswSelected;
        else
            M1_DutyA = (M1_Svpwm_T0/2)/M1_TswSelected;
            M1_DutyB = (M1_Svpwm_T1+M1_Svpwm_T2+M1_Svpwm_T0/2)/M1_TswSelected;
            M1_DutyC = (M1_Svpwm_T2+M1_Svpwm_T0/2)/M1_TswSelected;
        end
%         sectornumber = 3;
        return;
    end
    if (mod(M1_VoltageVectorAngleOptimum, 2*pi)<=4*pi/3)&&(mod(M1_VoltageVectorAngleOptimum, 2*pi)>=pi)  % sector 4
        M1_DutyA = (M1_Svpwm_T0/2)/M1_TswSelected;
        M1_DutyB = (M1_Svpwm_T1+M1_Svpwm_T0/2)/M1_TswSelected;
        M1_DutyC = (M1_Svpwm_T1+M1_Svpwm_T2+M1_Svpwm_T0/2)/M1_TswSelected;
%         sectornumber = 4;
        return;
    end
    if (mod(M1_VoltageVectorAngleOptimum, 2*pi)<=5*pi/3)&&(mod(M1_VoltageVectorAngleOptimum, 2*pi)>=4*pi/3)  % sector 5
        M1_DutyA = (M1_Svpwm_T2+M1_Svpwm_T0/2)/M1_TswSelected;
        M1_DutyB = (M1_Svpwm_T0/2)/M1_TswSelected;
        M1_DutyC = (M1_Svpwm_T1+M1_Svpwm_T2+M1_Svpwm_T0/2)/M1_TswSelected;
%         sectornumber = 5;
        return;
    end
    if (mod(M1_VoltageVectorAngleOptimum, 2*pi)<=2*pi)&&(mod(M1_VoltageVectorAngleOptimum, 2*pi)>=5*pi/3)  % sector 6
        M1_DutyA = (M1_Svpwm_T1+M1_Svpwm_T2+M1_Svpwm_T0/2)/M1_TswSelected;
        M1_DutyB = (M1_Svpwm_T0/2)/M1_TswSelected;
        M1_DutyC = (M1_Svpwm_T1+M1_Svpwm_T0/2)/M1_TswSelected;
%         sectornumber = 6;
        return;
    end
    
else %switching pulse
    M1_iqref = M1_iqref_prev;
    M1_Speed_Error = M1_Speed_Error_prev;
    M1_FswSelected = M1_FswSelected_prev;
    M1_DutyA = M1_DutyA_prev;
    M1_DutyB = M1_DutyB_prev;
    M1_DutyC = M1_DutyC_prev;
    M1_IqRipplePrediction = M1_IqRipplePrediction_prev;
end

== matlab function mpc_model_dual_module_tobecombined/MATLAB Function1 ==
  data: pulse input; inputwave input; outputwave output
function outputwave  = fcn(pulse, inputwave)

persistent state

if isempty(state)
state = 0;
end

if(pulse==1)
    state = state +1;
end

if(mod(state,2)==1)
    outputwave = inputwave;
    return;
end
if(mod(state,2)==0)
    outputwave = 1-inputwave;
    return;
end

outputwave = 5;

== matlab function mpc_model_dual_module_tobecombined/MATLAB Function2 ==
  data: pulse input; inputwave input; outputwave output
function outputwave  = fcn(pulse, inputwave)

persistent state

if isempty(state)
state = 0;
end

if(pulse==1)
    state = state +1;
end

if(mod(state,2)==1)
    outputwave = inputwave;
    return;
end
if(mod(state,2)==0)
    outputwave = 1-inputwave;
    return;
end

outputwave = 5;
